simulink model "sim_boganov_model"  (R2022b)
settings: Solver=FixedStepAuto  StartTime=2  StopTime=180  FixedStep=1  RelTol=1
values from neighbouring files (symbols this model uses):
  Gb = AP{1,2}    [zad2.m]    (also in zad2_gen.m)
  Ib = Ap{1,3}    [zad2.m]    (also in zad2_gen.m = AP{1,3})
  p2 = Pop(i,1)    [fitness.m]    (also in zad2.m = 0.0001016; zad2_gen.m = 0.000797976709042)
  Sg = Pop(i,3)    [fitness.m]    (also in zad2.m = 0.036105; zad2_gen.m = 0.0372645440805)
  Si = Pop(i,2)    [fitness.m]    (also in zad2.m = 0.13612; zad2_gen.m = 0.022114795308)
settings Model: Creator=DFUNDO  LastModifiedBy=DFUNDO

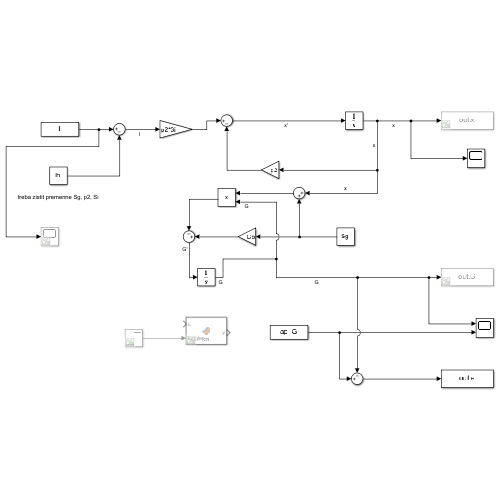
[thumbnail: Simulink's stored preview of the top-level diagram]
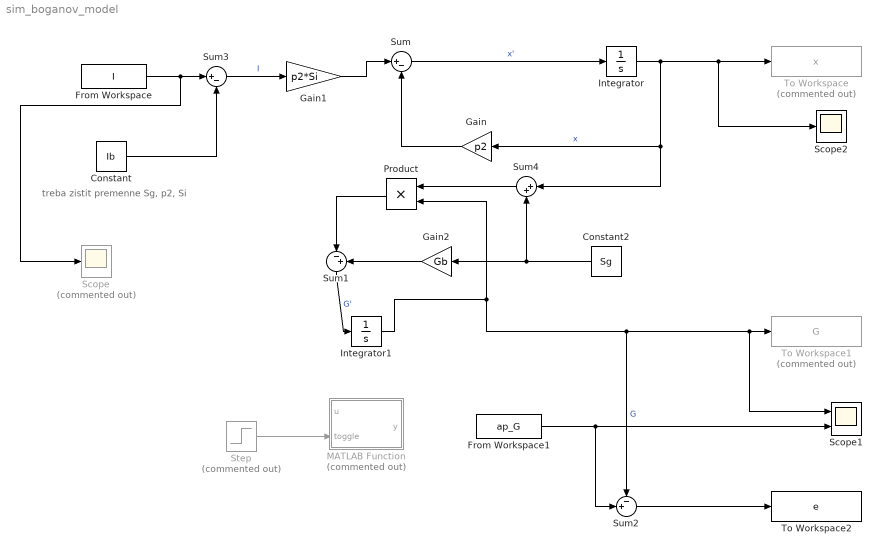
== system sim_boganov_model ==
  note: treba zistit premenne Sg, p2, Si
  Constant : Constant  Value=Ib
  Constant2 : Constant  Value=Sg
  From Workspace : FromWorkspace  VariableName=I
  From Workspace1 : FromWorkspace  VariableName=ap_G
  Gain : Gain  Gain=p2
  Gain1 : Gain  Gain=p2*Si
  Gain2 : Gain  Gain=Gb
  Integrator : Integrator
  Integrator1 : Integrator  InitialCondition=16.002790000000000
  MATLAB Function : MATLAB Function  Commented=on  TreatAsAtomicUnit=on
  Product : Product
  Scope : Scope  Commented=on
  Scope1 : Scope  NumInputPorts=2
  Scope2 : Scope
  Step : Step  Commented=on  Time=2  SampleTime=0
  Sum : Sum  Inputs=|+-
  Sum1 : Sum  Inputs=|-+
  Sum2 : Sum  Inputs=-+|
  Sum3 : Sum  Inputs=|+-
  Sum4 : Sum  Inputs=|++
  To Workspace : ToWorkspace  Commented=on  VariableName=x  SaveFormat=Timeseries  SampleTime=-1
  To Workspace1 : ToWorkspace  Commented=on  VariableName=G  SaveFormat=Timeseries  SampleTime=-1
  To Workspace2 : ToWorkspace  VariableName=e  SampleTime=-1
      settings: Save2DSignal=2-D array (concatenate along first dimension)
  wires:
  Sum/1 -> Integrator/1  "x'"
  Integrator/1 -> Scope2/1, To Workspace/1, Sum4/1, Gain/1  "x"
  Gain/1 -> Sum/2
  Gain1/1 -> Sum/1
  Sum3/1 -> Gain1/1  "I"
  Sum1/1 -> Integrator1/1  "G'"
  Integrator1/1 -> Scope1/1, To Workspace1/1, Sum2/1, Product/2  "G"
  Constant/1 -> Sum3/2
  From Workspace/1 -> Scope/1, Sum3/1
  Product/1 -> Sum1/1
  Constant2/1 -> Gain2/1, Sum4/2
  Sum4/1 -> Product/1
  Gain2/1 -> Sum1/2
  From Workspace1/1 -> Sum2/2, Scope1/2
  Sum2/1 -> To Workspace2/1
  Step/1 -> MATLAB Function/2(toggle)

== matlab function sim_boganov_model/MATLAB Function ==
  data: u input; y output; toggle input
function y = fcn(u,toggle)
if toggle
    y = u;
else
    y = 4.7038;
end
